simulink model "regular"  (Simulink 6.0)
settings: Solver=ode3  StartTime=0.0  StopTime=10.0  FixedStep=0.01  RelTol=1e-3
settings Model: LastModifiedBy=Administrator

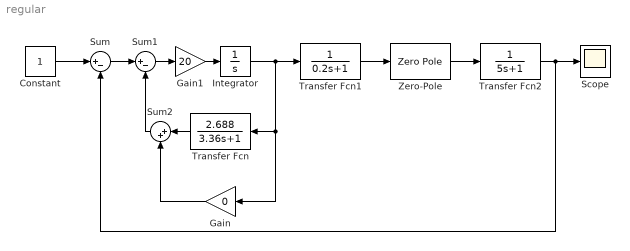
== system regular ==
  Constant : Constant
  Gain : Gain  Orientation=left  Gain=0
  Gain1 : Gain  Gain=20
  Integrator : Integrator
  Scope : Scope
  Sum : Sum  Inputs=|+-
  Sum1 : Sum  Inputs=|+-
  Sum2 : Sum  Orientation=left  Inputs=|++
  Transfer Fcn : TransferFcn  Orientation=left  Numerator=[2.688]  Denominator=[3.36 1]
  Transfer Fcn1 : TransferFcn  Denominator=[0.2 1]
  Transfer Fcn2 : TransferFcn  Denominator=[5 1]
  Zero-Pole : ZeroPole  Poles=[-2]  Gain=[-2]
  wires:
  Constant/1 -> Sum/1
  Sum/1 -> Sum1/1
  Integrator/1 -> Transfer Fcn1/1, Transfer Fcn/1, Gain/1
  Transfer Fcn1/1 -> Zero-Pole/1
  Zero-Pole/1 -> Transfer Fcn2/1
  Transfer Fcn2/1 -> Scope/1, Sum/2
  Gain/1 -> Sum2/2
  Transfer Fcn/1 -> Sum2/1
  Sum2/1 -> Sum1/2
  Gain1/1 -> Integrator/1
  Sum1/1 -> Gain1/1
